simulink model "Lab_10"  (R2018a)
settings: Solver=FixedStepDiscrete  StartTime=0.0  StopTime=Inf  RelTol=1e-3  EnableMultiTasking=on
libraries: dsparch4 x2
settings Model: Creator=The MathWorks, Inc.  LastModifiedBy=Colin Keenan
settings DataIOCC: LimitDataPoints=on  SaveFormat=Array  SignalLoggingName=logsOut
settings OptimizationCC: ExpressionDepthLimit=2147483647  InitFltsAndDblsToZero=on  EfficientMapNaN2IntZero=off  LifeSpan=inf
settings DebuggingCC: SaveWithParameterizedLinksMsg=none  UnderspecifiedInitializationDetection=Classic  MergeDetectMultiDrivingBlocksExec=none  CheckExecutionContextPreStartOutputMsg=on  CheckExecutionContextRuntimeOutputMsg=on  SolverPrmCheckMsg=warning  MultiTaskDSMMsg=warning  MultiTaskCondExecSysMsg=none  FcnCallInpInsideContextMsg=warning  StateNameClashWarn=warning  SFUnexpectedBacktrackingDiag=warning  SFNoUnconditionalDefaultTransitionDiag=warning  SFExecutionAtInitializationDiag=none
settings HardwareCC: ProdBitPerPointer=32  ProdBitPerSizeT=32  ProdBitPerPtrDiffT=32  ProdLargestAtomicFloat=None  ProdIntDivRoundTo=Undefined  ProdEndianess=Unspecified  ProdWordSize=32  ProdHWDeviceType=32-bit Generic
settings ModelReferenceCC: UpdateModelReferenceTargets=IfOutOfDate  PropagateSignalLabelsOutOfModel=off
settings CodeAppCC: StateflowObjectComments=on
settings GRTTargetCC: TargetFcnLib=ansi_tfl_tmw.mat  TargetLangStandard=C89/C90 (ANSI)  GeneratePreprocessorConditionals=Disable all  CombineOutputUpdateFcns=off  GRTInterface=on
settings ConfigComp: CovMetricSettings=dw  CovHtmlReporting=on  CovSaveCumulativeToWorkspaceVar=on  CovSaveSingleToWorkspaceVar=on  CovExternalEMLEnable=off

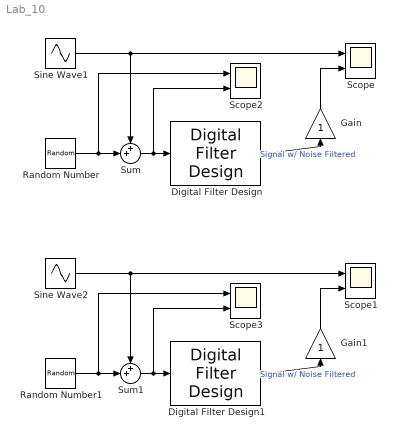
== system Lab_10 ==
  Digital Filter Design : dsparch4/Digital Filter Design  mwdsp_browser_bugfix_var=off
  Digital Filter Design1 : dsparch4/Digital Filter Design  mwdsp_browser_bugfix_var=off
  Gain : Gain
  Gain1 : Gain
  Random Number : RandomNumber  SampleTime=1/8000
  Random Number1 : RandomNumber  SampleTime=1/48000
  Scope{,1..3} (4 alike) : Scope  NumInputPorts=2
  Sine Wave1 : Sin  Frequency=2*pi*100  SampleTime=1/8000
  Sine Wave2 : Sin  Frequency=2*pi*500  SampleTime=1/48000
  Sum : Sum  Inputs=++|
  Sum1 : Sum  Inputs=++|
  wires:
  Sum/1 -> Scope2/2, Digital Filter Design/1
  Sine Wave1/1 -> Sum/1, Scope/1
  Digital Filter Design/1 -> Gain/1  "Signal w/ Noise Filtered"
  Random Number/1 -> Scope2/1, Sum/2
  Gain/1 -> Scope/2
  Sum1/1 -> Scope3/2, Digital Filter Design1/1
  Random Number1/1 -> Scope3/1, Sum1/2
  Digital Filter Design1/1 -> Gain1/1  "Signal w/ Noise Filtered"
  Sine Wave2/1 -> Sum1/1, Scope1/1
  Gain1/1 -> Scope1/2
